simulink model "trajectory_sim"  (R2022a)
settings: Solver=VariableStepAuto  StartTime=0.0  StopTime=1000.0  MaxStep=dt  RelTol=1e-3
values from neighbouring files (symbols this model uses):
  area = pi*0.42^2    (= 0.554176944093)    [rocket.m]    (also in rs_driverfile.m)
  burning_rate = mfuel/burn_time    (= 31.4003701419)    [rocket.m]    (also in rs_driverfile.m)
  Cd = [0.386 0.329 0.325 0.469 0.488 0.434 0.389 0.328 0.287 0.255 0.216      0.194 0.184 0.169 0.164 0.154 ]'    [rocket.m]    (also in rs_driverfile.m)
  D0 = 1.225    [planet.m]    (also in rs_driverfile.m)
  fthrust = 69.4*10^3    (= 69400)    [rocket.m]    (also in rs_driverfile.m)
  G = 6.67430*10^-11    (= 6.6743e-11)    [planet.m]    (also in rs_driverfile.m)
  H = 7640    [planet.m]    (also in rs_driverfile.m)
  hdg = 45*rad    (= 0.785398163397)    [rs_driver.m]    (also in rs_driverfile.m = 0)
  M = [0.1 0.5 0.8 1 1.2 1.5 2 2.5 3 3.5 4      4.5 5 5.5 6 6.5]'    [rocket.m]    (also in rs_driverfile.m)
  mearth = 5.9722*10^24    (= 5.9722e+24)    [rs_driverfile.m]
  mfuel = 1018    [rocket.m]    (also in rs_driverfile.m)
  mrocket = 1261    [rocket.m]    (also in rs_driverfile.m = 1361)
  nozzle_area = pi*0.34^2    (= 0.363168110755)    [rocket.m]    (also in rs_driverfile.m)
  P0 = 1.01325*10^5    (= 101325)    [planet.m]    (also in rs_driverfile.m)
  pitch = 0*rad    (= 0)    [rs_driver.m]    (also in rs_driverfile.m = 0.785398163397)
  r_earth = 6.3781*10^6    (= 6378100)    [rs_driverfile.m]
  v0 = 8612.6    [rs_driver.m]    (also in rs_driverfile.m = 0)
  x0 = [ ... (first row only)    [rs_driver.m]    (also in rs_driverfile.m = 0)
  y0 = 0    [rs_driverfile.m]
  z0 = 0    [rs_driverfile.m]
undefined symbols (not defined in the file or in its folder): magnitude
libraries: simulink x5
settings Model: Creator=mitch  LastModifiedBy=mitch
settings DataIOCC: ReturnWorkspaceOutputs=off

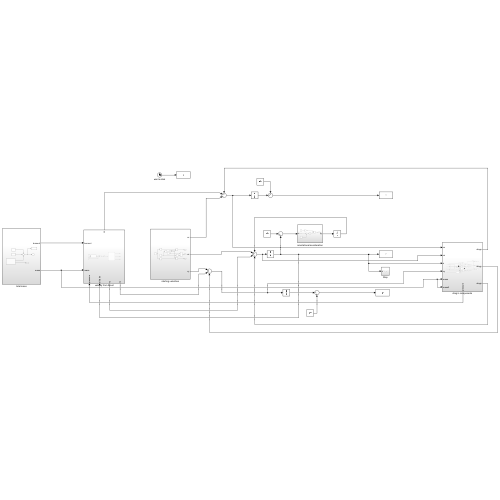
[thumbnail: Simulink's stored preview of the top-level diagram]
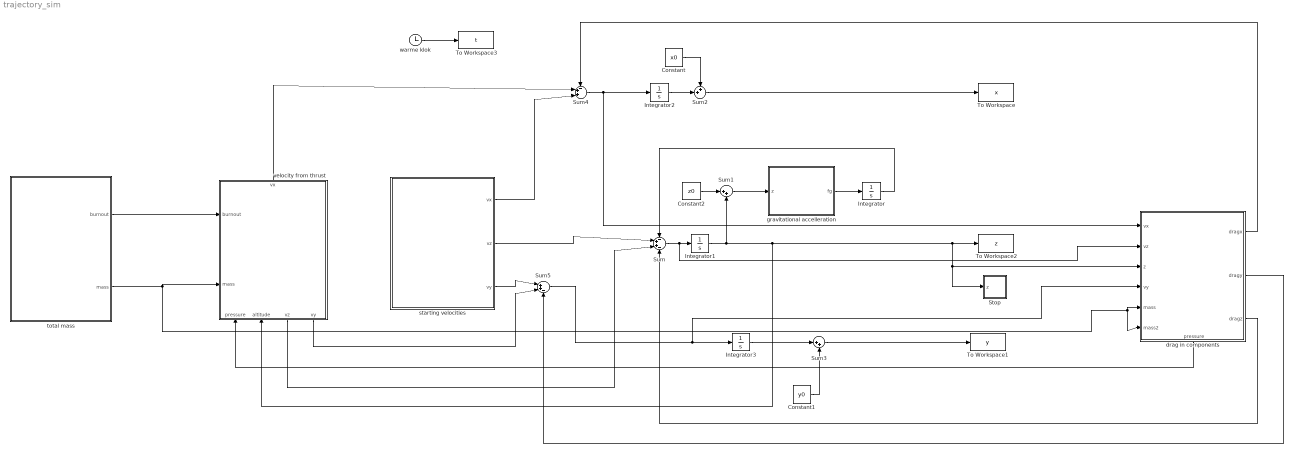
== system trajectory_sim ==
  Constant : Constant  Value=x0
  Constant1 : Constant  Value=y0
  Constant2 : Constant  Value=z0
  Integrator{,1..3} (4 alike) : Integrator
  Stop : Subsystem
  Sum : Sum  Inputs=-++-
  Sum1 : Sum  Inputs=|++
  Sum2 : Sum  Inputs=++|
  Sum3 : Sum  Inputs=|++
  Sum4 : Sum  Inputs=-++|
  Sum5 : Sum  Inputs=|++-
  To Workspace : ToWorkspace  VariableName=x  SampleTime=-1
  To Workspace1 : ToWorkspace  VariableName=y  SampleTime=-1
  To Workspace2 : ToWorkspace  VariableName=z  SampleTime=-1
  To Workspace3 : ToWorkspace  VariableName=t  SampleTime=-1
  drag in components : Subsystem
      settings: PortSchema="{\"entries\":[{\"content\":{\"sides\":[{\"content\":{\"connectorIds\":[\"In1\",\"In2\",\"In3\",\"In4\",\"In5\",\"In6\"]},\"type\":\"ConnectorPlacement.EquallySpacedRectSide\",\"uuid\":\"270dc5b8-5525-47cd-975a-4958e02966d3\"},{\"content\":{\"connectorIds\":[\"Out1\",\"Out2\",\"Out3\"],\"side\":\"RIGHT\"},\"type\":\"ConnectorPlacement.EquallySpacedRectSide\",\"uuid\":\"3fa3747e-ccec-4eab-8472-d73208bed964\"},{\"content\":{\"connectorIds\":[],\"side\":\"TOP\"},\"type\":\"ConnectorPlacement.EquallySpacedRectSide\",\"uuid\":\"51e6e8ff-8d60-4d27-80b7-dcbe5b12a41c\"},{\"content\":{\"connectorIds\":[\"Out4\"],\"side\":\"BOTTOM\"},\"type\":\"ConnectorPlacement.EquallySpacedRectSide\",\"uuid\":\"057fab17-4ba9-4fa5-8b65-fe355dab7313\"}]},\"type\":\"ConnectorPlacement.EquallySpacedConnector\",\"uuid\":\"0b03f533-b71d-47fe-a33a-bac65d9138e6\"}],\"packageUris\":[\"http://schema.mathworks.com/mf0/Connector/R2020b\"],\"version\":\"1.0\"}"
  gravitational accelleration : Subsystem
  starting velocities : Subsystem
  total mass : Subsystem
  velocity from thrust : Subsystem
      settings: PortSchema="{\"entries\":[{\"content\":{\"sides\":[{\"content\":{\"connectorIds\":[\"In1\",\"In2\"]},\"type\":\"ConnectorPlacement.EquallySpacedRectSide\",\"uuid\":\"d4dbb746-52d6-4045-8ea1-207ff2e3e58c\"},{\"content\":{\"connectorIds\":[],\"side\":\"RIGHT\"},\"type\":\"ConnectorPlacement.EquallySpacedRectSide\",\"uuid\":\"1ffc5929-0dda-49c4-bcef-0917812487df\"},{\"content\":{\"connectorIds\":[\"Out3\"],\"side\":\"TOP\"},\"type\":\"ConnectorPlacement.EquallySpacedRectSide\",\"uuid\":\"4f5e6482-bb4e-4c79-8aed-4c633bc645bd\"},{\"content\":{\"connectorIds\":[\"In3\",\"In4\",\"Out1\",\"Out2\"],\"side\":\"BOTTOM\"},\"type\":\"ConnectorPlacement.EquallySpacedRectSide\",\"uuid\":\"3b572149-e164-4a06-99d0-85ce38077b62\"}]},\"type\":\"ConnectorPlacement.EquallySpacedConnector\",\"uuid\":\"5475df72-feae-4ad9-b564-185b0fab10d9\"}],\"packageUris\":[\"http://schema.mathworks.com/mf0/Connector/R2020b\"],\"version\":\"1.0\"}"
  warme klok : Clock
  wires:
  gravitational accelleration/1(fg) -> Integrator/1
  Sum/1 -> drag in components/2(vz), Integrator1/1
  Sum2/1 -> To Workspace/1
  Integrator1/1 -> velocity from thrust/4(altitude), Stop/1(z), drag in components/3(z), To Workspace2/1, Sum1/2
  Sum1/1 -> gravitational accelleration/1(z)
  Sum3/1 -> To Workspace1/1
  Integrator2/1 -> Sum2/2
  Constant/1 -> Sum2/1
  Integrator3/1 -> Sum3/1
  Constant2/1 -> Sum1/1
  Constant1/1 -> Sum3/2
  Integrator/1 -> Sum/1
  starting velocities/2(vz) -> Sum/2
  Sum4/1 -> drag in components/1(vx), Integrator2/1
  starting velocities/1(vx) -> Sum4/3
  Sum5/1 -> drag in components/4(vy), Integrator3/1
  starting velocities/3(vy) -> Sum5/1
  warme klok/1 -> To Workspace3/1
  total mass/1(burnout) -> velocity from thrust/1(burnout)
  total mass/2(mass) -> drag in components/6(mass2), drag in components/5(mass), velocity from thrust/2(mass)
  velocity from thrust/3(vx) -> Sum4/2
  velocity from thrust/1(vz) -> Sum/3
  velocity from thrust/2(vy) -> Sum5/2
  drag in components/2(dragy) -> Sum5/3
  drag in components/1(dragx) -> Sum4/1
  drag in components/3(dragz) -> Sum/4
  drag in components/4(pressure) -> velocity from thrust/3(pressure)

== system trajectory_sim/Stop ==
  z : Inport
  Compare To Zero : simulink/Logic and Bit Operations/Compare To Zero  relop=<  OutDataTypeStr=boolean
  Stop Simulation : Stop
  wires:
  Compare To Zero/1 -> Stop Simulation/1
  z/1 -> Compare To Zero/1

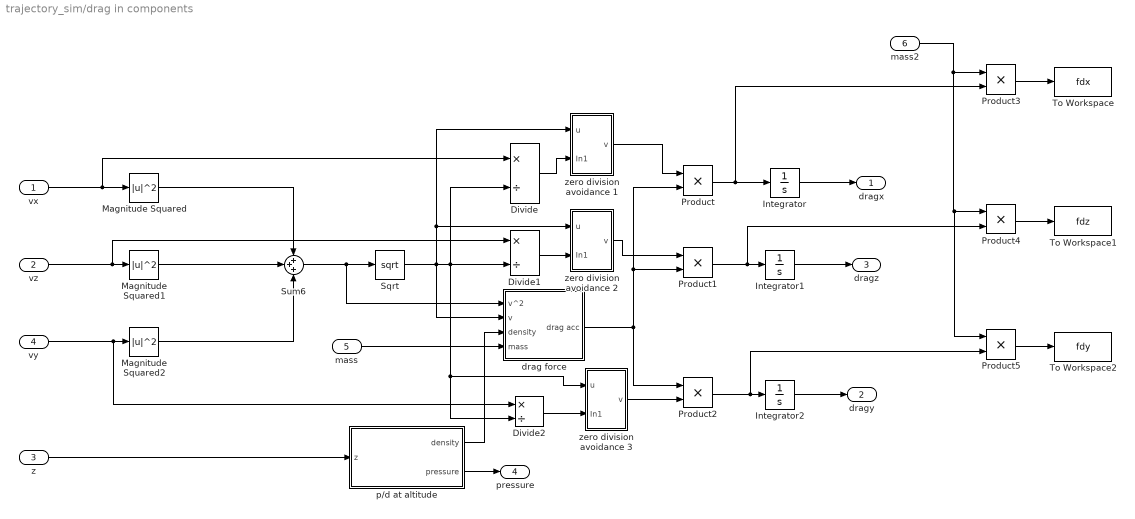
== system trajectory_sim/drag in components ==
  vx : Inport
  vz : Inport  Port=2
  z : Inport  Port=3
  vy : Inport  Port=4
  mass : Inport  Port=5
  mass2 : Inport  Port=6
  Divide : Product  Inputs=*/
  Divide1 : Product  Inputs=*/
  Divide2 : Product  Inputs=*/
  Integrator : Integrator
  Integrator1 : Integrator
  Integrator2 : Integrator
  Magnitude Squared : Math  Operator=magnitude^2
  Magnitude Squared1 : Math  Operator=magnitude^2
  Magnitude Squared2 : Math  Operator=magnitude^2
  Product{,1..5} (6 alike) : Product
  Sqrt : Sqrt
  Sum6 : Sum  Inputs=+++
  To Workspace : ToWorkspace  VariableName=fdx  SampleTime=-1
  To Workspace1 : ToWorkspace  VariableName=fdz  SampleTime=-1
  To Workspace2 : ToWorkspace  VariableName=fdy  SampleTime=-1
  drag force : Subsystem
  p/d at altitude : Subsystem
  zero division avoidance 1 : Subsystem
  zero division avoidance 2 : Subsystem
  zero division avoidance 3 : Subsystem
  dragx : Outport
  dragy : Outport  Port=2
  dragz : Outport  Port=3
  pressure : Outport  Port=4
  wires:
  vx/1 -> Divide/1, Magnitude Squared/1
  Sum6/1 -> drag force/1(v^2), Sqrt/1
  vz/1 -> Divide1/1, Magnitude Squared1/1
  Magnitude Squared2/1 -> Sum6/3
  vy/1 -> Divide2/1, Magnitude Squared2/1
  Magnitude Squared1/1 -> Sum6/2
  Magnitude Squared/1 -> Sum6/1
  Sqrt/1 -> zero division avoidance 1/1(u), zero division avoidance 2/1(u), drag force/2(v), Divide/2, Divide2/2, zero division avoidance 3/1(u), Divide1/2
  z/1 -> p/d at altitude/1(z)
  p/d at altitude/1(density) -> drag force/3(density)
  drag force/1(drag acc) -> Product/2, Product1/2, Product2/1
  mass/1 -> drag force/4(mass)
  Product/1 -> Product3/2, Integrator/1
  Product1/1 -> Product4/2, Integrator1/1
  Product2/1 -> Product5/2, Integrator2/1
  Integrator/1 -> dragx/1
  Integrator1/1 -> dragz/1
  Integrator2/1 -> dragy/1
  Divide/1 -> zero division avoidance 1/2(In1)
  zero division avoidance 1/1(v) -> Product/1
  Divide1/1 -> zero division avoidance 2/2(In1)
  zero division avoidance 2/1(v) -> Product1/1
  zero division avoidance 3/1(v) -> Product2/2
  Divide2/1 -> zero division avoidance 3/2(In1)
  p/d at altitude/2(pressure) -> pressure/1
  Product3/1 -> To Workspace/1
  Product4/1 -> To Workspace1/1
  Product5/1 -> To Workspace2/1
  mass2/1 -> Product5/1, Product4/1, Product3/1

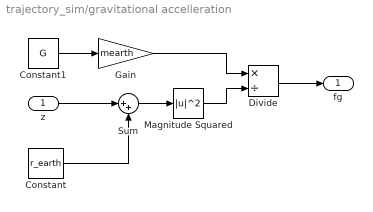
== system trajectory_sim/gravitational accelleration ==
  z : Inport
  Constant : Constant  Value=r_earth
  Constant1 : Constant  Value=G
  Divide : Product  Inputs=*/
  Gain : Gain  Gain=mearth
  Magnitude Squared : Math  Operator=magnitude^2
  Sum : Sum  Inputs=|++
  fg : Outport
  wires:
  Constant1/1 -> Gain/1
  Divide/1 -> fg/1
  Gain/1 -> Divide/1
  z/1 -> Sum/1
  Constant/1 -> Sum/2
  Sum/1 -> Magnitude Squared/1
  Magnitude Squared/1 -> Divide/2

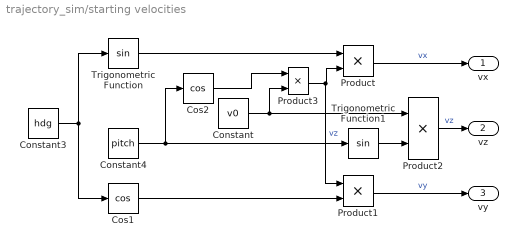
== system trajectory_sim/starting velocities ==
  Constant : Constant  Value=v0
  Constant3 : Constant  Value=hdg
  Constant4 : Constant  Value=pitch
  Cos1 : Trigonometry  Operator=cos
  Cos2 : Trigonometry  Operator=cos
  Product{,1..3} (4 alike) : Product
  Trigonometric Function : Trigonometry
  Trigonometric Function1 : Trigonometry
  vx : Outport
  vz : Outport  Port=2
  vy : Outport  Port=3
  wires:
  Constant/1 -> Product3/2, Product2/1
  Product2/1 -> vz/1  "vz"
  Product1/1 -> vy/1  "vy"
  Trigonometric Function/1 -> Product/1
  Constant3/1 -> Cos1/1, Trigonometric Function/1
  Product/1 -> vx/1  "vx"
  Cos2/1 -> Product3/1
  Constant4/1 -> Cos2/1, Trigonometric Function1/1
  Trigonometric Function1/1 -> Product2/2
  Product3/1 -> Product1/1, Product/2  "vz"
  Cos1/1 -> Product1/2

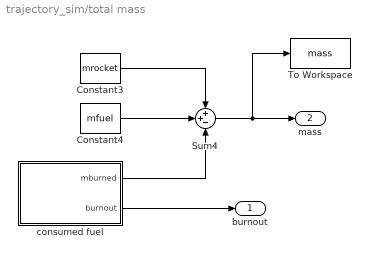
== system trajectory_sim/total mass ==
  Constant3 : Constant  Value=mrocket
  Constant4 : Constant  Value=mfuel
  Sum4 : Sum  Inputs=++-
  To Workspace : ToWorkspace  VariableName=mass  SampleTime=-1
  consumed fuel : Subsystem
  burnout : Outport
  mass : Outport  Port=2
  wires:
  Sum4/1 -> To Workspace/1, mass/1
  Constant4/1 -> Sum4/2
  consumed fuel/1(mburned) -> Sum4/3
  Constant3/1 -> Sum4/1
  consumed fuel/2(burnout) -> burnout/1

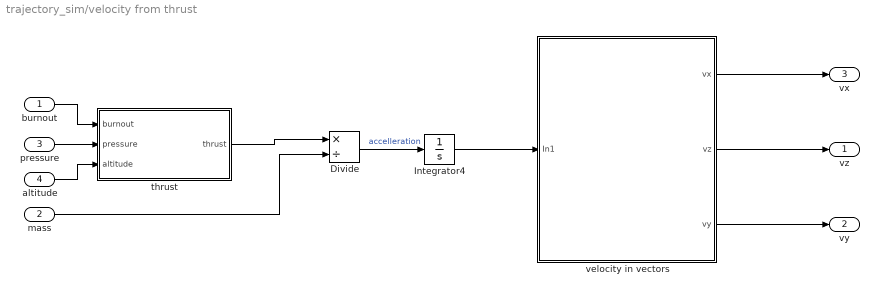
== system trajectory_sim/velocity from thrust ==
  burnout : Inport
  mass : Inport  Port=2
  pressure : Inport  Port=3
  altitude : Inport  Port=4
  Divide : Product  Inputs=*/
  Integrator4 : Integrator
  thrust : Subsystem
  velocity in vectors : Subsystem
  vz : Outport
  vy : Outport  Port=2
  vx : Outport  Port=3
  wires:
  velocity in vectors/3(vy) -> vy/1
  mass/1 -> Divide/2
  thrust/1(thrust) -> Divide/1
  Divide/1 -> Integrator4/1  "accelleration"
  Integrator4/1 -> velocity in vectors/1(In1)
  velocity in vectors/2(vz) -> vz/1
  burnout/1 -> thrust/1(burnout)
  velocity in vectors/1(vx) -> vx/1
  pressure/1 -> thrust/2(pressure)
  altitude/1 -> thrust/3(altitude)

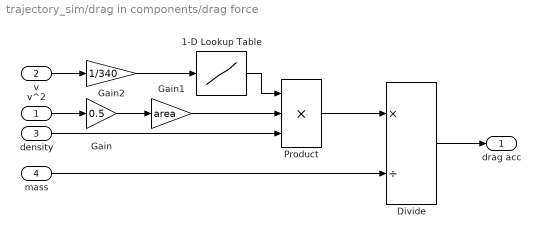
== system trajectory_sim/drag in components/drag force ==
  v^2 : Inport
  v : Inport  Port=2
  density : Inport  Port=3
  mass : Inport  Port=4
  1-D Lookup Table : Lookup_n-D  NumberOfTableDimensions=1  BreakpointsForDimension1=M  Table=Cd  InternalRulePriority=Speed  RndMeth=Simplest
  Divide : Product  Inputs=*/
  Gain : Gain  Gain=0.5
  Gain1 : Gain  Gain=area
  Gain2 : Gain  Gain=1/340
  Product : Product  Inputs=3
  drag acc : Outport
  wires:
  Gain1/1 -> Product/2
  v^2/1 -> Gain/1
  Gain2/1 -> 1-D Lookup Table/1
  1-D Lookup Table/1 -> Product/1
  v/1 -> Gain2/1
  density/1 -> Product/3
  Gain/1 -> Gain1/1
  Product/1 -> Divide/1
  Divide/1 -> drag acc/1
  mass/1 -> Divide/2

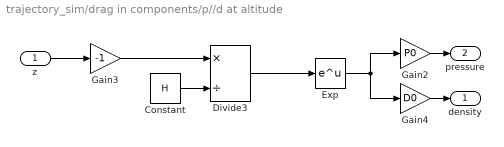
== system trajectory_sim/drag in components/p//d at altitude ==
  z : Inport
  Constant : Constant  Value=H
  Divide3 : Product  Inputs=*/
  Exp : Math
  Gain2 : Gain  Gain=P0
  Gain3 : Gain  Gain=-1
  Gain4 : Gain  Gain=D0
  density : Outport
  pressure : Outport  Port=2
  wires:
  Gain3/1 -> Divide3/1
  Constant/1 -> Divide3/2
  Gain4/1 -> density/1
  Exp/1 -> Gain2/1, Gain4/1
  Gain2/1 -> pressure/1
  Divide3/1 -> Exp/1
  z/1 -> Gain3/1

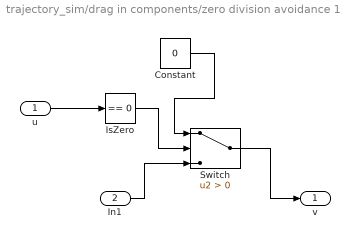
== system trajectory_sim/drag in components/zero division avoidance 1 ==
  u : Inport
  In1 : Inport  Port=2
  Constant : Constant  Value=0
  IsZero : simulink/Logic and Bit Operations/Compare To Zero  relop===  OutDataTypeStr=boolean
  Switch : Switch  Criteria=u2 > Threshold  SaturateOnIntegerOverflow=off  InputSameDT=off
  v : Outport
  wires:
  Switch/1 -> v/1
  Constant/1 -> Switch/1
  IsZero/1 -> Switch/2
  u/1 -> IsZero/1
  In1/1 -> Switch/3

== system trajectory_sim/drag in components/zero division avoidance 2 ==
  u : Inport
  In1 : Inport  Port=2
  Constant : Constant  Value=0
  IsZero : simulink/Logic and Bit Operations/Compare To Zero  relop===  OutDataTypeStr=boolean
  Switch : Switch  Criteria=u2 > Threshold  SaturateOnIntegerOverflow=off  InputSameDT=off
  v : Outport
  wires:
  Switch/1 -> v/1
  Constant/1 -> Switch/1
  IsZero/1 -> Switch/2
  u/1 -> IsZero/1
  In1/1 -> Switch/3

== system trajectory_sim/drag in components/zero division avoidance 3 ==
  u : Inport
  In1 : Inport  Port=2
  Constant : Constant  Value=0
  IsZero : simulink/Logic and Bit Operations/Compare To Zero  relop===  OutDataTypeStr=boolean
  Switch : Switch  Criteria=u2 > Threshold  SaturateOnIntegerOverflow=off  InputSameDT=off
  v : Outport
  wires:
  Switch/1 -> v/1
  Constant/1 -> Switch/1
  IsZero/1 -> Switch/2
  u/1 -> IsZero/1
  In1/1 -> Switch/3

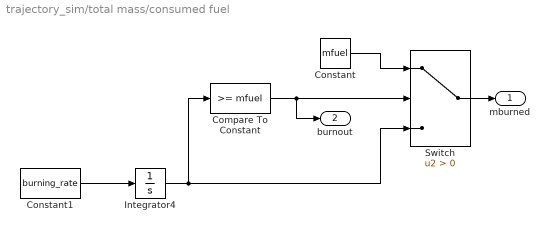
== system trajectory_sim/total mass/consumed fuel ==
  Compare To Constant : simulink/Logic and Bit Operations/Compare To Constant  relop=>=  const=mfuel  OutDataTypeStr=boolean
  Constant : Constant  Value=mfuel
  Constant1 : Constant  Value=burning_rate
  Integrator4 : Integrator
  Switch : Switch  Criteria=u2 > Threshold  SaturateOnIntegerOverflow=off  InputSameDT=off
  mburned : Outport
  burnout : Outport  Port=2
  wires:
  Integrator4/1 -> Compare To Constant/1, Switch/3
  Compare To Constant/1 -> burnout/1, Switch/2
  Switch/1 -> mburned/1
  Constant/1 -> Switch/1
  Constant1/1 -> Integrator4/1

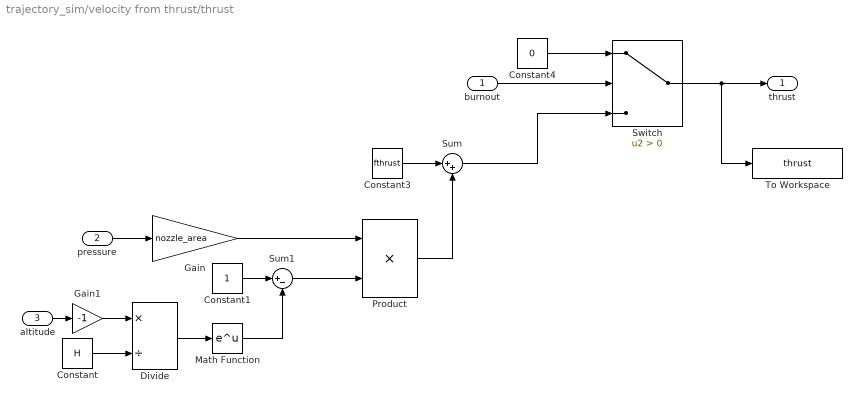
== system trajectory_sim/velocity from thrust/thrust ==
  burnout : Inport
  pressure : Inport  Port=2
  altitude : Inport  Port=3
  Constant : Constant  Value=H
  Constant1 : Constant
  Constant3 : Constant  Value=fthrust
  Constant4 : Constant  Value=0
  Divide : Product  Inputs=*/
  Gain : Gain  Gain=nozzle_area
  Gain1 : Gain  Gain=-1
  Math Function : Math
  Product : Product
  Sum : Sum  Inputs=|++
  Sum1 : Sum  Inputs=|+-
  Switch : Switch  Criteria=u2 > Threshold  SaturateOnIntegerOverflow=off  InputSameDT=off
  To Workspace : ToWorkspace  VariableName=thrust  SampleTime=-1
  thrust : Outport
  wires:
  Switch/1 -> To Workspace/1, thrust/1
  burnout/1 -> Switch/2
  Constant4/1 -> Switch/1
  Constant3/1 -> Sum/1
  pressure/1 -> Gain/1
  altitude/1 -> Gain1/1
  Gain1/1 -> Divide/1
  Constant/1 -> Divide/2
  Divide/1 -> Math Function/1
  Math Function/1 -> Sum1/2
  Constant1/1 -> Sum1/1
  Gain/1 -> Product/1
  Sum1/1 -> Product/2
  Product/1 -> Sum/2
  Sum/1 -> Switch/3

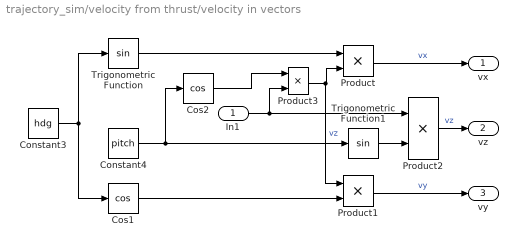
== system trajectory_sim/velocity from thrust/velocity in vectors ==
  In1 : Inport
  Constant3 : Constant  Value=hdg
  Constant4 : Constant  Value=pitch
  Cos1 : Trigonometry  Operator=cos
  Cos2 : Trigonometry  Operator=cos
  Product{,1..3} (4 alike) : Product
  Trigonometric Function : Trigonometry
  Trigonometric Function1 : Trigonometry
  vx : Outport
  vz : Outport  Port=2
  vy : Outport  Port=3
  wires:
  Constant3/1 -> Cos1/1, Trigonometric Function/1
  Product2/1 -> vz/1  "vz"
  Trigonometric Function/1 -> Product/1
  Cos1/1 -> Product1/2
  Constant4/1 -> Cos2/1, Trigonometric Function1/1
  Product/1 -> vx/1  "vx"
  Product1/1 -> vy/1  "vy"
  Trigonometric Function1/1 -> Product2/2
  In1/1 -> Product3/2, Product2/1
  Cos2/1 -> Product3/1
  Product3/1 -> Product1/1, Product/2  "vz"
